simulink model "s0414"  (Simulink 7.0)
settings: Solver=ode3  SolverMode=SingleTasking  StartTime=0.0  StopTime=900  FixedStep=1  MaxStep=1  RelTol=1e-3  AbsTol=1e-6
values from neighbouring files (symbols this model uses):
  Gsnen = Gs.den{1}    [m0404Bsp.m]
  Gszae = Gs.num{1}    [m0404Bsp.m]
  Kpr = 10    [m0108d.m]    (also in m0109b.m = 1; m0113c.m; m0404Bsp.m = 3)
  wdach_ = wdach    (= 1)    [m0404Bsp.m]
  zdach_ = zdach    (= 1)    [m0404Bsp.m]
undefined symbols (not defined in the file or in its folder): Kir
settings Model: Creator=froriep  LastModifiedBy=froriep
settings DataIOCC: LimitDataPoints=off  SaveOutput=off  SaveTime=off
settings OptimizationCC: BooleanDataType=off
settings DebuggingCC: SaveWithParameterizedLinksMsg=none  SignalResolutionControl=TryResolveAllWithWarning  SolverPrmCheckMsg=none  MultiTaskDSMMsg=warning  MultiTaskCondExecSysMsg=none  StrictBusMsg=None
settings HardwareCC: TargetUnknown=on
settings RTWCC: IncludeERTFirstTime=on

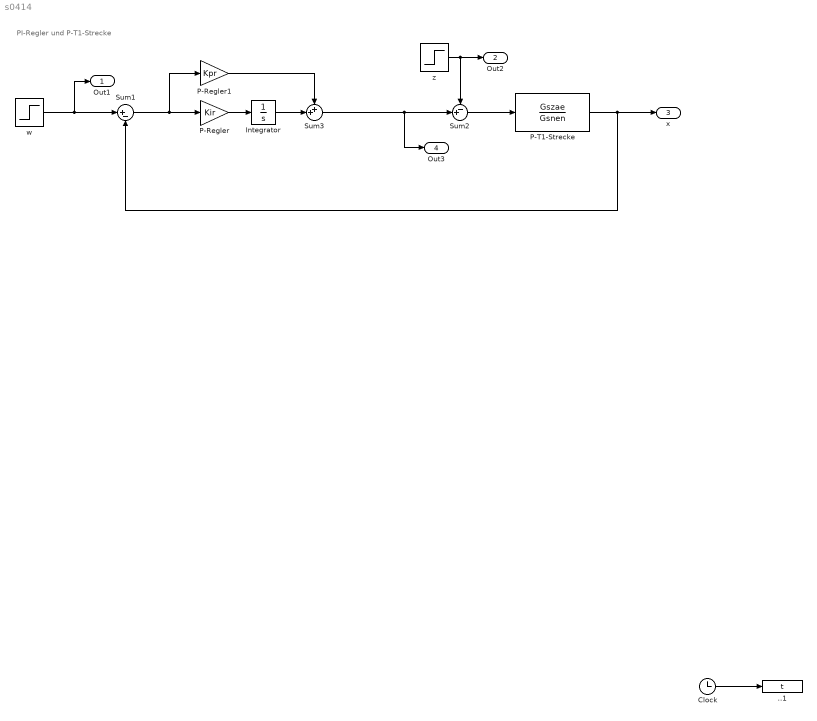
== system s0414 ==
  note: PI-Regler und P-T1-Strecke
  ..1 : ToWorkspace  VariableName=t  SaveFormat=Array
  Clock : Clock
      settings: Decimation=10
  Integrator : Integrator
  P-Regler : Gain  Gain=Kir  ParameterDataType=sfix(16)  ParameterScaling=2^0  OutDataType=sfix(16)  OutScaling=2^0
  P-Regler1 : Gain  Gain=Kpr  ParameterDataType=sfix(16)  ParameterScaling=2^0  OutDataType=sfix(16)  OutScaling=2^0
  P-T1-Strecke : TransferFcn  Numerator=Gszae  Denominator=Gsnen
  Sum1 : Sum  Inputs=|+-  SaturateOnIntegerOverflow=on  InputSameDT=on
  Sum2 : Sum  Inputs=-+|  SaturateOnIntegerOverflow=on  InputSameDT=on
  Sum3 : Sum  Inputs=++|  SaturateOnIntegerOverflow=on  InputSameDT=on
  w : Step  After=wdach_  SampleTime=0
  z : Step  After=zdach_  SampleTime=0
  Out1 : Outport  OutDataType=sfix(16)  OutScaling=2^0
  Out2 : Outport  Port=2  OutDataType=sfix(16)  OutScaling=2^0
  x : Outport  Port=3  OutDataType=sfix(16)  OutScaling=2^0
  Out3 : Outport  Port=4  OutDataType=sfix(16)  OutScaling=2^0
  wires:
  z/1 -> Sum2/1, Out2/1
  w/1 -> Sum1/1, Out1/1
  Sum1/1 -> P-Regler/1, P-Regler1/1
  Clock/1 -> ..1/1
  P-T1-Strecke/1 -> Sum1/2, x/1
  Sum2/1 -> P-T1-Strecke/1
  P-Regler1/1 -> Sum3/1
  P-Regler/1 -> Integrator/1
  Integrator/1 -> Sum3/2
  Sum3/1 -> Sum2/2, Out3/1
